simulink model "kalman_control_simulink"  (R2020a)
settings: Solver=VariableStepAuto  StartTime=0.0  StopTime=0  RelTol=1e-3
values from neighbouring files (symbols this model uses):
  C_meas = [    DYN.C       ,      eye(2)    ]    [Kalman_control.m]
  control_gain = 1    [Kalman_control.m]
  dt = 0.001    [Filter_color_clean.m]    (also in Filter_white.m = 0.0001; Kalman_control.m = 0.000244140625; Steady_state_Kalman.m = 0.000244140625; doubsus.m = obj.dt)
  highselector = [1,     0,    0,  0,  0,  0]    [Kalman_control.m]
  lowselector = [0,     1,    0,  0,  0,  0]    [Kalman_control.m]
libraries: cstblocks x7
settings Model: OrderedModelArguments=off  Creator=eddbonilla  LastModifiedBy=eddbonilla

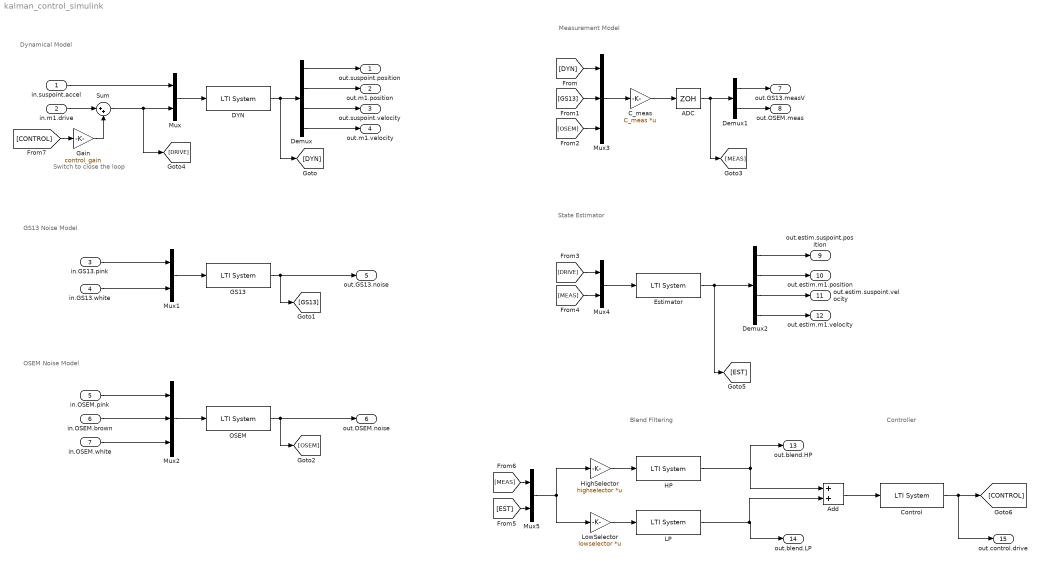
== system kalman_control_simulink ==
  note: Dynamical Model
  note: GS13 Noise Model
  note: OSEM Noise Model
  note: Measurement Model
  note: State Estimator
  note: Blend Filtering
  note: Controller
  note: Switch to
      | close the loop
  in.suspoint.accel : Inport
  in.m1.drive : Inport  Port=2
  in.GS13.pink : Inport  Port=3
  in.GS13.white : Inport  Port=4
  in.OSEM.pink : Inport  Port=5
  in.OSEM.brown : Inport  Port=6
  in.OSEM.white : Inport  Port=7
  ADC : ZeroOrderHold  SampleTime=dt
  Add : Sum
  C_meas : Gain  Gain=C_meas  Multiplication=Matrix(K*u)
  Control : cstblocks/LTI System  sys=control  IC=[]
  DYN : cstblocks/LTI System  sys=dyn  IC=[]
  Demux : Demux
  Demux1 : Demux  Outputs=2
  Demux2 : Demux
  Estimator : cstblocks/LTI System  sys=estimator  IC=[]
  GS13 : cstblocks/LTI System  sys=gs13  IC=[]
  Gain : Gain  Gain=control_gain
  HP : cstblocks/LTI System  sys=hp  IC=[]
  HighSelector : Gain  Gain=highselector  Multiplication=Matrix(K*u)
  LP : cstblocks/LTI System  sys=lp  IC=[]
  LowSelector : Gain  Gain=lowselector  Multiplication=Matrix(K*u)
  Mux{,1,4..5} (4 alike) : Mux  Inputs=2
  Mux2 : Mux  Inputs=3
  Mux3 : Mux  Inputs=3
  OSEM : cstblocks/LTI System  sys=osem  IC=[]
  Sum : Sum  Inputs=|++
  out.suspoint.position : Outport
  out.m1.position : Outport  Port=2
  out.suspoint.velocity : Outport  Port=3
  out.m1.velocity : Outport  Port=4
  out.GS13.noise : Outport  Port=5
  out.OSEM.noise : Outport  Port=6
  out.GS13.measV : Outport  Port=7
  out.OSEM.meas : Outport  Port=8
  out.estim.suspoint.position : Outport  Port=9
  out.estim.m1.position : Outport  Port=10
  out.estim.suspoint.velocity : Outport  Port=11
  out.estim.m1.velocity : Outport  Port=12
  out.blend.HP : Outport  Port=13
  out.blend.LP : Outport  Port=14
  out.control.drive : Outport  Port=15
  wires:
  Mux/1 -> DYN/1
  in.suspoint.accel/1 -> Mux/1
  DYN/1 -> [DYN], Demux/1
  Demux/4 -> out.m1.velocity/1
  Demux/1 -> out.suspoint.position/1
  Demux/2 -> out.m1.position/1
  Demux/3 -> out.suspoint.velocity/1
  GS13/1 -> [GS13], out.GS13.noise/1
  Mux1/1 -> GS13/1
  in.GS13.pink/1 -> Mux1/1
  in.GS13.white/1 -> Mux1/2
  in.OSEM.white/1 -> Mux2/3
  in.OSEM.brown/1 -> Mux2/2
  Mux2/1 -> OSEM/1
  in.OSEM.pink/1 -> Mux2/1
  OSEM/1 -> [OSEM], out.OSEM.noise/1
  C_meas/1 -> ADC/1
  Mux3/1 -> C_meas/1
  [DYN] -> Mux3/1
  [GS13] -> Mux3/2
  [OSEM] -> Mux3/3
  ADC/1 -> [MEAS], Demux1/1
  Demux1/1 -> out.GS13.measV/1
  Demux1/2 -> out.OSEM.meas/1
  Mux4/1 -> Estimator/1
  [DRIVE] -> Mux4/1
  [MEAS] -> Mux4/2
  Estimator/1 -> [EST], Demux2/1
  Demux2/2 -> out.estim.m1.position/1
  Demux2/1 -> out.estim.suspoint.position/1
  Demux2/4 -> out.estim.m1.velocity/1
  [MEAS] -> Mux5/1
  [EST] -> Mux5/2
  Mux5/1 -> HighSelector/1, LowSelector/1
  HighSelector/1 -> HP/1
  LowSelector/1 -> LP/1
  HP/1 -> Add/1, out.blend.HP/1
  Control/1 -> out.control.drive/1, [CONTROL]
  LP/1 -> Add/2, out.blend.LP/1
  Demux2/3 -> out.estim.suspoint.velocity/1
  Add/1 -> Control/1
  in.m1.drive/1 -> Sum/1
  Sum/1 -> [DRIVE], Mux/2
  [CONTROL] -> Gain/1
  Gain/1 -> Sum/2
